simulink library "alfa_window_in"  (R2018b)
settings: Solver=ode45  StartTime=0.0  StopTime=10.0  RelTol=1e-3  EnableMultiTasking=on
settings Model: Creator=lena.frank  LastModifiedBy=goettsche
settings DataIOCC: LimitDataPoints=on  SaveFormat=Array  SignalLoggingSaveFormat=ModelDataLogs
settings OptimizationCC: ExpressionDepthLimit=2147483647  LifeSpan=inf
settings DebuggingCC: UnderspecifiedInitializationDetection=Classic  MergeDetectMultiDrivingBlocksExec=none  SolverPrmCheckMsg=warning  FcnCallInpInsideContextMsg=warning  StateNameClashWarn=warning  SFUnexpectedBacktrackingDiag=warning  SFNoUnconditionalDefaultTransitionDiag=warning  SFExecutionAtInitializationDiag=none
settings HardwareCC: ProdBitPerPointer=32  ProdBitPerSizeT=32  ProdBitPerPtrDiffT=32  ProdLargestAtomicFloat=None  ProdIntDivRoundTo=Undefined  ProdEndianess=Unspecified  ProdWordSize=32  ProdHWDeviceType=32-bit Generic
settings ModelReferenceCC: PropagateSignalLabelsOutOfModel=off
settings SFSimCC: SimUseLocalCustomCode=off
settings RTWCC: RTWUseLocalCustomCode=off
settings CodeAppCC: StateflowObjectComments=on
settings GRTTargetCC: TargetLangStandard=C89/C90 (ANSI)  CombineOutputUpdateFcns=off  GRTInterface=on
settings ConfigComp: CovMetricSettings=dw  CovHtmlReporting=on  CovSaveCumulativeToWorkspaceVar=on  CovSaveSingleToWorkspaceVar=on  CovExternalEMLEnable=off

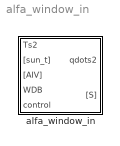
== system alfa_window_in ==
  alfa_window_in : Subsystem  mask(ALFA){type_glazing=double glazing normal, gvalue=0.7, tauzero=0.8, emission_in=1, wallsurface=1, frame=0.1, numlayer=2, shad_type=No shading, tau_shad=0.01, bli_a=0.05, bli_b=1, bli_c=0.05, bli_d=0.05, bli_alpha=90, bli_refl=0.2}
      mask prompts: type_glazing "glazing type"; gvalue "Energy transmission by sunlight (g-value) 0..1"; tauzero "transmittance in visible range of the sunlight [0..1]"; emission_in "Longwave emissivity (0..1)"; wallsurface "Surface of the window (with frame) in m²"; frame "Share of the frame on the surface (0...1)"; numlayer "Number of glass panes"; shad_type "shading type [no Shading/exterior/interior]"; tau_shad "solar transmittance of shading element [0..1]"; bli_a "a  Depth of blind blades [m]"; bli_b "b heigth of blind blades [m]"; bli_c "c distance of "b" to back end of blind blade [m]"; bli_d "d offset between blind blades [m]"; bli_refl "optical reflectance of blind surface [0..1]"
      mask help:
      | Convective and radiative heat transfer at the INDOOR SURFACE OF A VERTICAL WINDOW with 1-4 layers (each 3 ... 8 mm thick).
      |
      | Ts  : temperature of window surface, °C,
      | [sun_t]  : sun data (incidence angle, direct and diffuse radiation
      |     at tilted window surface),
      | [AIV]  : conditions of zone node,
      | qdots  : specific heat flow into window construction, W/m^2,
      | qdot_abs : specific irradiation absorption within window
      |     construction,  W/m^2,
      | [S]  : heat and air flow to zone node.
      mask Help: web(fullfile(path_carnot('help'),'alfa_window_in.html'),'-helpbrowser')
      mask TypeOptions type_glazing: double glazing normal | double glazing  thermal insulation | double glazing combi 73/41 | double glazing combi 50/24 | triple glazing normal | triple glazing  thermal insulation
      mask TypeOptions tauzero: Subsystem/tau(0)/Gain
      mask TypeOptions shad_type: No shading | Exterior Screen | Interior Screen | Venetian Blind

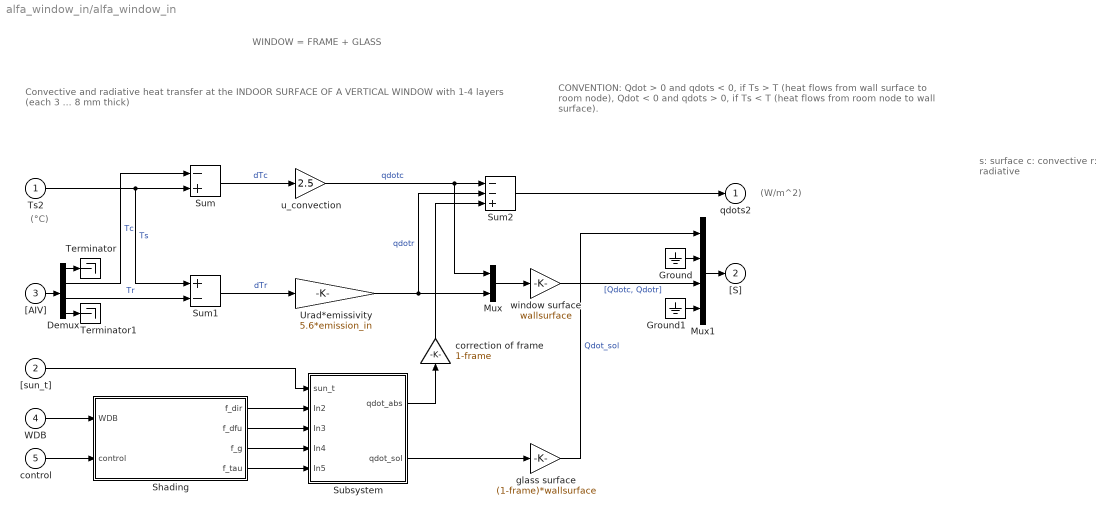
== system alfa_window_in/alfa_window_in ==
  note: (°C)
  note: Convective and radiative heat transfer at the INDOOR SURFACE OF A VERTICAL WINDOW
      | with 1-4 layers (each 3 ... 8 mm thick)
  note: WINDOW = FRAME + GLASS
  note: s: surface
      | c: convective
      | r: radiative
  note: CONVENTION:
      | Qdot > 0 and qdots < 0, if Ts > T (heat flows from wall surface to room node),
      | Qdot < 0 and qdots > 0, if Ts < T (heat flows from room node to wall surface).
  note: (W/m^2)
  Ts2 : Inport
  "[sun_t]" : Inport  Port=2
  "[AIV]" : Inport  Port=3
  WDB : Inport  Port=4
  control : Inport  Port=5
  " glass surface" : Gain  Gain=(1-frame)*wallsurface  SaturateOnIntegerOverflow=on  OutDataTypeStr=Inherit: Same as input  ParamDataTypeStr=Inherit: Same as input
  Demux : Demux  Outputs=[1 1 1 6]
      settings: DisplayOption=none
  Ground : Ground
  Ground1 : Ground
  Mux : Mux  Inputs=2
  Mux1 : Mux  Inputs=[1 5 2 5]
  Shading : Subsystem
  Subsystem : Subsystem
  Sum : Sum  Inputs=-+  InputSameDT=on  SaturateOnIntegerOverflow=on  OutDataTypeStr=Inherit: Same as first input
  Sum1 : Sum  Inputs=+-  InputSameDT=on  SaturateOnIntegerOverflow=on  OutDataTypeStr=Inherit: Same as first input
  Sum2 : Sum  Inputs=--+  InputSameDT=on  SaturateOnIntegerOverflow=on  OutDataTypeStr=Inherit: Same as first input
  Terminator : Terminator
  Terminator1 : Terminator
  Urad*emissivity : Gain  Gain=5.6*emission_in  SaturateOnIntegerOverflow=on  OutDataTypeStr=Inherit: Same as input  ParamDataTypeStr=Inherit: Same as input
  correction of frame : Gain  Gain=1-frame
  u_convection : Gain  Gain=2.5  SaturateOnIntegerOverflow=on  OutDataTypeStr=Inherit: Same as input  ParamDataTypeStr=Inherit: Same as input
  window surface : Gain  Gain=wallsurface  SaturateOnIntegerOverflow=on  OutDataTypeStr=Inherit: Same as input  ParamDataTypeStr=Inherit: Same as input
  qdots2 : Outport  VectorParamsAs1DForOutWhenUnconnected=off
  "[S]" : Outport  Port=2  VectorParamsAs1DForOutWhenUnconnected=off
  wires:
  Demux/3 -> Sum1/2  "Tr"
  Sum/1 -> u_convection/1  "dTc"
  Demux/2 -> Sum/1  "Tc"
  window surface/1 -> Mux1/3  "[Qdotc, Qdotr]"
  " glass surface"/1 -> Mux1/1  "Qdot_sol"
  u_convection/1 -> Sum2/1, Mux/1  "qdotc"
  Urad*emissivity/1 -> Mux/2, Sum2/2  "qdotr"
  Ts2/1 -> Sum1/1, Sum/2  "Ts"
  Sum1/1 -> Urad*emissivity/1  "dTr"
  Mux/1 -> window surface/1
  Demux/1 -> Terminator/1
  "[AIV]"/1 -> Demux/1
  Demux/4 -> Terminator1/1
  Sum2/1 -> qdots2/1
  Mux1/1 -> "[S]"/1
  Ground/1 -> Mux1/2
  Ground1/1 -> Mux1/4
  control/1 -> Shading/2(control)
  WDB/1 -> Shading/1(WDB)
  "[sun_t]"/1 -> Subsystem/1(sun_t)
  Shading/1(f_dir) -> Subsystem/2(In2)
  Shading/2(f_dfu) -> Subsystem/3(In3)
  Shading/3(f_g) -> Subsystem/4(In4)
  Shading/4(f_tau) -> Subsystem/5(In5)
  Subsystem/1(qdot_abs) -> correction of frame/1
  Subsystem/2(qdot_sol) -> " glass surface"/1
  correction of frame/1 -> Sum2/3

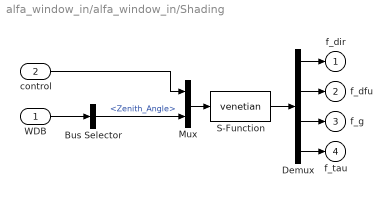
== system alfa_window_in/alfa_window_in/Shading ==
  WDB : Inport
  control : Inport  Port=2
  Bus Selector : BusSelector  OutputSignals=Zenith_Angle
  Demux : Demux
  Mux : Mux  Inputs=2
  S-Function : S-Function  FunctionName=venetian  Parameters=bli_a, bli_b, bli_c, bli_d, bli_alpha, bli_refl, shad_type, type_glazing, tau_shad  SFunctionDeploymentMode=off  EnableBusSupport=off
  f_dir : Outport  VectorParamsAs1DForOutWhenUnconnected=off
  f_dfu : Outport  Port=2  VectorParamsAs1DForOutWhenUnconnected=off
  f_g : Outport  Port=3  VectorParamsAs1DForOutWhenUnconnected=off
  f_tau : Outport  Port=4  VectorParamsAs1DForOutWhenUnconnected=off
  wires:
  Demux/4 -> f_tau/1
  Demux/3 -> f_g/1
  Demux/2 -> f_dfu/1
  Demux/1 -> f_dir/1
  S-Function/1 -> Demux/1
  Mux/1 -> S-Function/1
  control/1 -> Mux/1
  Bus Selector/1 -> Mux/2  "<Zenith_Angle>"
  WDB/1 -> Bus Selector/1

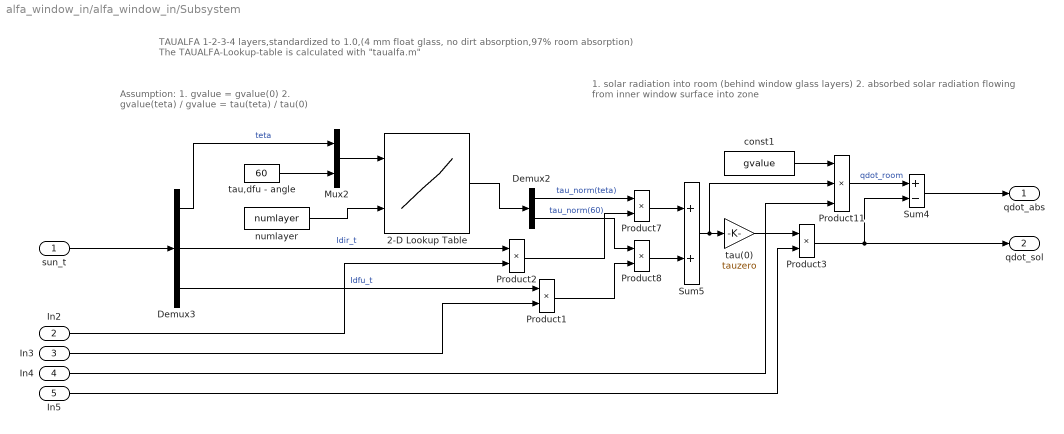
== system alfa_window_in/alfa_window_in/Subsystem ==
  note: Assumption:
      | 1. gvalue = gvalue(0)
      | 2. gvalue(teta) / gvalue = tau(teta) / tau(0)
  note: TAUALFA 1-2-3-4 layers,standardized to 1.0,(4 mm float glass, no dirt absorption,97% room absorption)
      | The TAUALFA-Lookup-table is calculated with "taualfa.m"
  note: 1. solar radiation into room (behind window glass layers)
      | 2. absorbed solar radiation flowing from inner window surface into zone
  sun_t : Inport
  In2 : Inport  Port=2
  In3 : Inport  Port=3
  In4 : Inport  Port=4
  In5 : Inport  Port=5
  2-D Lookup Table : Lookup_n-D  BreakpointsForDimension1=[0:10:90]  BreakpointsForDimension2=[1:4]  Table=[1.0000 1.0000 1.0000 1.0000; 0.9996 0.9991 0.9987 0.9983; 0.9979 0.9961 0.9945 0.9929; 0.9937 0.9894 0.9861 0.9836; 0.9839 0.9753 0.9704 0.9680; 0.9608 0.9438 0.9365 0.9361; 0.9061 0.8679 0.8484 0.8413; 0.7755 0.6821 0.6182 0.5717; 0.4807 0.3277 0.2324 0.1688; 0 0 0 0]  InternalRulePriority=Speed  RndMeth=Simplest  InputSameDT=on
  Demux2 : Demux  Outputs=2
      settings: DisplayOption=none
  Demux3 : Demux  Outputs=3
      settings: DisplayOption=none
  Mux2 : Mux  Inputs=2
  Product{1..3,7..8} (5 alike) : Product  InputSameDT=on  RndMeth=Zero  SaturateOnIntegerOverflow=on  OutDataTypeStr=Inherit: Same as first input
  Product11 : Product  Inputs=3  InputSameDT=on  RndMeth=Zero  SaturateOnIntegerOverflow=on  OutDataTypeStr=Inherit: Same as first input
  Sum4 : Sum  Inputs=+-  InputSameDT=on  SaturateOnIntegerOverflow=on  OutDataTypeStr=Inherit: Same as first input
  Sum5 : Sum  InputSameDT=on  SaturateOnIntegerOverflow=on  OutDataTypeStr=Inherit: Same as first input
  const1 : Constant  Value=gvalue
  numlayer : Constant  Value=numlayer
  tau(0) : Gain  Gain=tauzero  SaturateOnIntegerOverflow=on  OutDataTypeStr=Inherit: Same as input  ParamDataTypeStr=Inherit: Same as input
  tau,dfu - angle : Constant  Value=60
  qdot_abs : Outport  VectorParamsAs1DForOutWhenUnconnected=off
  qdot_sol : Outport  Port=2  VectorParamsAs1DForOutWhenUnconnected=off
  wires:
  Product1/1 -> Product8/2
  2-D Lookup Table/1 -> Demux2/1
  sun_t/1 -> Demux3/1
  In3/1 -> Product1/2
  Mux2/1 -> 2-D Lookup Table/1
  Demux3/1 -> Mux2/1  "teta"
  Demux3/2 -> Product2/1  "Idir_t"
  const1/1 -> Product11/1
  Demux3/3 -> Product1/1  "Idfu_t"
  tau,dfu - angle/1 -> Mux2/2
  tau(0)/1 -> Product3/1
  Product2/1 -> Product7/2
  Product8/1 -> Sum5/2
  Product3/1 -> qdot_sol/1, Sum4/2
  Sum5/1 -> tau(0)/1, Product11/2
  Product7/1 -> Sum5/1
  Product11/1 -> Sum4/1  "qdot_room"
  In4/1 -> Product11/3
  Demux2/1 -> Product7/1  "tau_norm(teta)"
  numlayer/1 -> 2-D Lookup Table/2
  Demux2/2 -> Product8/1  "tau_norm(60)"
  Sum4/1 -> qdot_abs/1
  In2/1 -> Product2/2
  In5/1 -> Product3/2
